simulink model "ans2"  (R2024b)
settings: Solver=VariableStepAuto  StartTime=0.0  StopTime=1  RelTol=1e-3
settings Model: Creator=32602  LastModifiedBy=32602

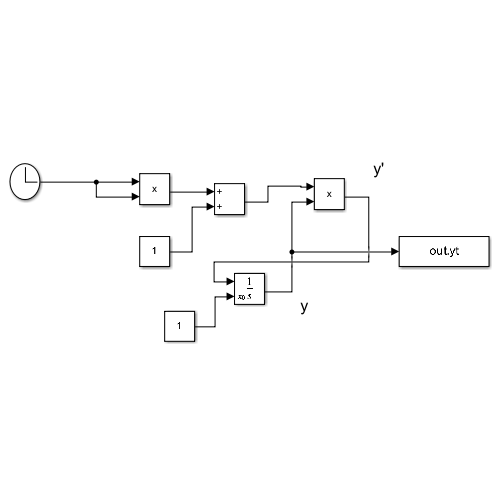
[thumbnail: Simulink's stored preview of the top-level diagram]
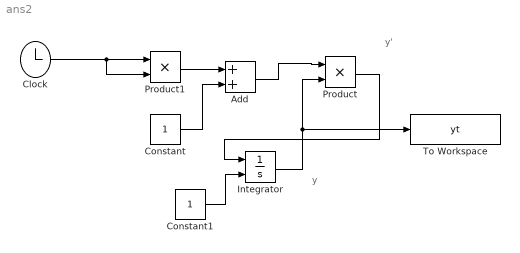
== system ans2 ==
  note: y
  note: y'
  Add : Sum
  Clock : Clock
  Constant : Constant
  Constant1 : Constant
  Integrator : Integrator  InitialConditionSource=external  InitialCondition=1
  Product : Product
  Product1 : Product
  To Workspace : ToWorkspace  VariableName=yt  SaveFormat=Timeseries  SampleTime=-1
  wires:
  Clock/1 -> Product1/2, Product1/1
  Constant/1 -> Add/2
  Product1/1 -> Add/1
  Integrator/1 -> Product/2, To Workspace/1
  Add/1 -> Product/1
  Product/1 -> Integrator/1
  Constant1/1 -> Integrator/2
